simulink model "lqg_mod_flexible_beam"  (R2018b)
settings: Solver=ode23t  StartTime=0.0  StopTime=60  MaxStep=1e-3  RelTol=1e-3
values from neighbouring files (symbols this model uses):
  A = [1.1269   -0.4940    0.1129, ... (first row only)    [kalman_filter_ex_discr.m]    (also in kalman_filter_example.m = [0 1 0;0 0 1;1 0 0]; lqg_example.m = [0 1 0;0 0 1;1 0 0]; lqg_rolling_mill.m = Pdes.a; lqr_inverted_pendulum.m = [0      1              0           0)
  B = [-0.3832 ... (first row only)    [kalman_filter_ex_discr.m]    (also in kalman_filter_example.m = [0.3 1;0 1;-0.3 0.9]; lqg_example.m = [0.3 1;0 1;-0.3 0.9]; lqg_rolling_mill.m = Pdes.b(:,1:2); lqr_inverted_pendulum.m = [     0)
  C = [1 0 0]    [kalman_filter_ex_discr.m]    (also in kalman_filter_example.m = [1.9 1.3 1]; lqg_example.m = [1.9 1.3 1]; lqg_rolling_mill.m = Pdes.c(3:4,:); lqr_inverted_pendulum.m = [1 0 0 0)
  D = 0    [kalman_filter_ex_discr.m]    (also in kalman_filter_example.m = [0.53 -0.61]; lqg_example.m = [0.53 -0.61]; lqg_rolling_mill.m = Pdes.d(3:4,1:2); lqr_inverted_pendulum.m = [0)
undefined symbols (not defined in the file or in its folder): Kf, Kr
settings Model: Creator=mircea  LastModifiedBy=mircea

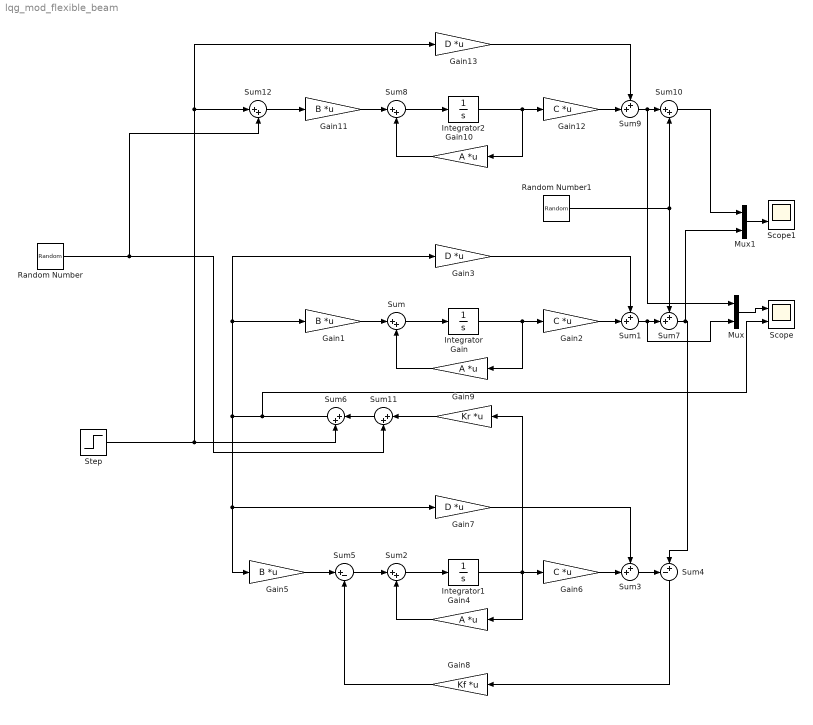
== system lqg_mod_flexible_beam ==
  Gain : Gain  Gain=A  Multiplication=Matrix(K*u) (u vector)
  Gain1 : Gain  Gain=B  Multiplication=Matrix(K*u) (u vector)
  Gain10 : Gain  Gain=A  Multiplication=Matrix(K*u) (u vector)
  Gain11 : Gain  Gain=B  Multiplication=Matrix(K*u) (u vector)
  Gain12 : Gain  Gain=C  Multiplication=Matrix(K*u) (u vector)
  Gain13 : Gain  Gain=D  Multiplication=Matrix(K*u) (u vector)
  Gain2 : Gain  Gain=C  Multiplication=Matrix(K*u) (u vector)
  Gain3 : Gain  Gain=D  Multiplication=Matrix(K*u) (u vector)
  Gain4 : Gain  Gain=A  Multiplication=Matrix(K*u) (u vector)
  Gain5 : Gain  Gain=B  Multiplication=Matrix(K*u) (u vector)
  Gain6 : Gain  Gain=C  Multiplication=Matrix(K*u) (u vector)
  Gain7 : Gain  Gain=D  Multiplication=Matrix(K*u) (u vector)
  Gain8 : Gain  Gain=Kf  Multiplication=Matrix(K*u) (u vector)
  Gain9 : Gain  Gain=Kr  Multiplication=Matrix(K*u) (u vector)
  Integrator : Integrator
  Integrator1 : Integrator
  Integrator2 : Integrator
  Mux : Mux  Inputs=2
  Mux1 : Mux  Inputs=2
  Random Number : RandomNumber  SampleTime=0.01
  Random Number1 : RandomNumber  Variance=0.01  SampleTime=0.001
  Scope : Scope  NumInputPorts=2
  Scope1 : Scope  NumInputPorts=2
  Step : Step  Time=0  SampleTime=0
  Sum{,2,6,8,10..12} (7 alike) : Sum  Inputs=|++
  Sum{1,3,7,9} (4 alike) : Sum  Inputs=++|
  Sum4 : Sum  Inputs=-+|
  Sum5 : Sum  Inputs=|+-
  wires:
  Mux/1 -> Scope/1
  Sum/1 -> Integrator/1
  Gain/1 -> Sum/2
  Integrator/1 -> Gain2/1, Gain/1
  Gain1/1 -> Sum/1
  Gain2/1 -> Sum1/2
  Gain3/1 -> Sum1/1
  Gain6/1 -> Sum3/2
  Sum2/1 -> Integrator1/1
  Gain7/1 -> Sum3/1
  Gain4/1 -> Sum2/2
  Integrator1/1 -> Gain9/1, Gain6/1, Gain4/1
  Sum3/1 -> Sum4/1
  Sum4/1 -> Gain8/1
  Sum5/1 -> Sum2/1
  Gain5/1 -> Sum5/1
  Gain8/1 -> Sum5/2
  Gain12/1 -> Sum9/2
  Gain10/1 -> Sum8/2
  Integrator2/1 -> Gain12/1, Gain10/1
  Step/1 -> Sum12/1, Gain13/1, Sum6/2
  Sum8/1 -> Integrator2/1
  Gain13/1 -> Sum9/1
  Gain11/1 -> Sum8/1
  Sum9/1 -> Mux/1, Sum10/1
  Sum11/1 -> Sum6/1
  Gain9/1 -> Sum11/1
  Sum7/1 -> Mux1/2, Sum4/2
  Sum1/1 -> Mux/2, Sum7/2
  Sum12/1 -> Gain11/1
  Random Number/1 -> Sum11/2, Sum12/2
  Random Number1/1 -> Sum7/1, Sum10/2
  Sum6/1 -> Scope/2, Gain7/1, Gain5/1, Gain3/1, Gain1/1
  Mux1/1 -> Scope1/2
  Sum10/1 -> Mux1/1
